simulink model "C28069_LLC_ePWM_V8_230307_PhaeShiftWorking"  (R2022b)
settings: Solver=FixedStepAuto  StartTime=0.0  StopTime=10  RelTol=1e-3  EnableMultiTasking=on
model workspace (MAT data in the model file):
  Comp_DAC = 512
undefined symbols (not defined in the file or in its folder): Down, GPTRIP1SEL, GPTRIP2SEL, PWM_Control, PWM_Gen, PWM_Gen1, SCI_A_Transmit, SCI_A_Transmit_Current_Suffix, SCI_A_Transmit_Duty_Suffix, SCI_A_Transmit_Freq_Suffix, SCI_A_Transmit_OVPFlag_Suffix, SCI_A_Transmit_PFC_Suffix, SCI_A_Transmit_SS_Suffix, SCI_A_Transmit_TBPHS_Suffix, SCI_A_Transmit_VADC_Suffix, SCI_A_Transmit_VAvg_Suffix, SCI_A_Transmit_VBAT_Suffix, SCI_A_Transmit_VBATRef_Suffix, SCI_A_Transmit_Vo_Suffix, TZ1, TZ2, u1, Up
libraries: c2802xlib x92, c280xlib x39, simulink x36, c2000lib x1
(part 3 of 18)

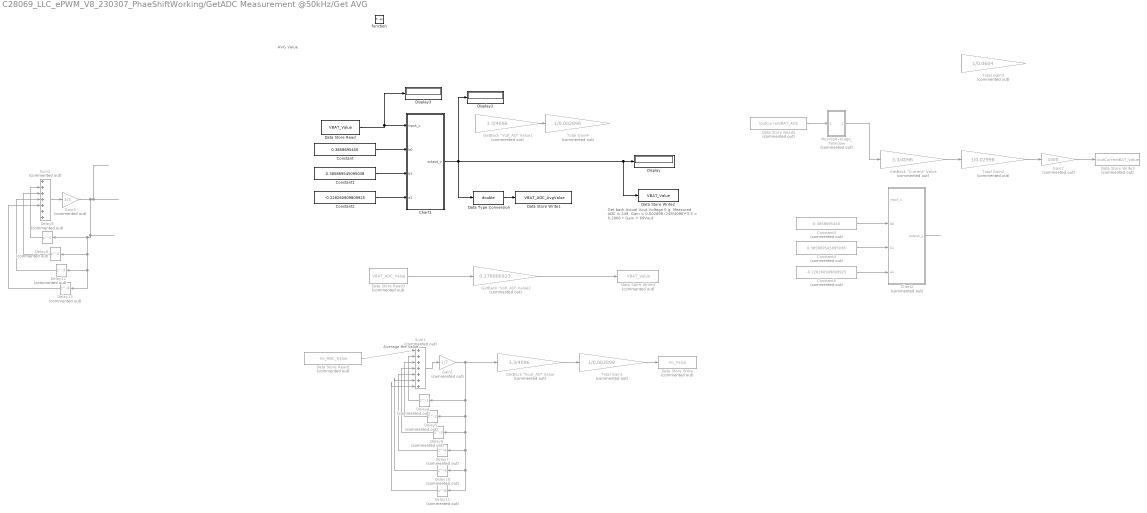
== system C28069_LLC_ePWM_V8_230307_PhaeShiftWorking/GetADC Measurement @50kHz/Get AVG ==
  note: AVG Value
  note: Average the value
  note: Get back Actual Vout Voltage
      | E.g.
      | Measured ADC is 249, Gain = 0.002898
      | (249/4096)*3.3 = 0.2006 * Gain
      | = 69Vout
  function : TriggerPort  TriggerType=function-call  VariantControl=(inherit)
  Chart1 : Stateflow chart  TreatAsAtomicUnit=on
  Chart2 : Stateflow chart  Commented=on  TreatAsAtomicUnit=on
  Constant : Constant  Value=0.3858695450
  Constant1 : Constant  Value=0.385869545095038
  Constant2 : Constant  Value=-0.228260909809925
  Constant3 : Constant  Commented=on  Value=0.3858695450
  Constant4 : Constant  Commented=on  Value=0.385869545095038
  Constant5 : Constant  Commented=on  Value=-0.228260909809925
  Data Store Read : DataStoreRead  DataStoreName=VBAT_Value  IndexOptions=Index vector (dialog)  Indices=1  OutputSizes=1
  Data Store Read1 : DataStoreRead  Commented=on  DataStoreName=Vo_ADC_Value  IndexOptions=Index vector (dialog)  Indices=1  OutputSizes=1
  Data Store Read2 : DataStoreRead  Commented=on  DataStoreName=IoutCurrentBAT_ADC  IndexOptions=Index vector (dialog)  Indices=1  OutputSizes=1
  Data Store Read3 : DataStoreRead  Commented=on  DataStoreName=VBAT_ADC_Value  IndexOptions=Index vector (dialog)  Indices=1  OutputSizes=1
  Data Store Write : DataStoreWrite  Commented=on  DataStoreName=Vo_Value  IndexOptions=Index vector (dialog)  Indices=1  OutputSizes=1
  Data Store Write1 : DataStoreWrite  DataStoreName=VBAT_ADC_AvgValue  IndexOptions=Index vector (dialog)  Indices=1  OutputSizes=1
  Data Store Write2 : DataStoreWrite  DataStoreName=VBAT_Value  IndexOptions=Index vector (dialog)  Indices=1  OutputSizes=1
  Data Store Write3 : DataStoreWrite  Commented=on  DataStoreName=IoutCurrentBAT_Value  IndexOptions=Index vector (dialog)  Indices=1  OutputSizes=1
  Data Store Write4 : DataStoreWrite  Commented=on  DataStoreName=VBAT_Value  IndexOptions=Index vector (dialog)  Indices=1  OutputSizes=1
  Data Type Conversion : DataTypeConversion  OutDataTypeStr=double  SaturateOnIntegerOverflow=off  RndMeth=Floor
  Delay10 : Delay  Commented=on  DelayLength=5
  Delay11 : Delay  Commented=on  DelayLength=6
  Delay12 : Delay  Commented=on  DelayLength=3
  Delay13 : Delay  Commented=on  DelayLength=4
  Delay4 : Delay  Commented=on  DelayLength=1
  Delay5 : Delay  Commented=on
  Delay6 : Delay  Commented=on  DelayLength=3
  Delay7 : Delay  Commented=on  DelayLength=4
  Delay8 : Delay  Commented=on  DelayLength=1
  Delay9 : Delay  Commented=on
  Display : Display
      settings: Decimation=2
  Display2 : Display
  Display3 : Display
  Gain1 : Gain  Commented=on  Gain=1/7  OutDataTypeStr=uint16
  Gain2 : Gain  Commented=on  Gain=1000
  Gain3 : Gain  Commented=on  Gain=1/5  OutDataTypeStr=uint16
  "GetBack \"Current\" Value" : Gain  Commented=on  Gain=3.3/4096  OutDataTypeStr=double
  "GetBack \"Volt_AD\" Value1" : Gain  Commented=on  Gain=3.3/4096  OutDataTypeStr=double
  "GetBack \"Volt_AD\" Value2" : Gain  Commented=on  Gain=0.278006923  OutDataTypeStr=double
  "GetBack \"Vout_AD\" Value" : Gain  Commented=on  Gain=3.3/4096  OutDataTypeStr=double
  MovingAverage_7Window : Subsystem  Commented=on
  Sum1 : Sum  Commented=on  Inputs=|+++++++
  Sum2 : Sum  Commented=on  Inputs=|+++++++
  Total Gain1 : Gain  Commented=on  Gain=1/0.002898  OutDataTypeStr=double
  Total Gain2 : Gain  Commented=on  Gain=1/0.02998  OutDataTypeStr=double
  Total Gain3 : Gain  Commented=on  Gain=1/0.0604  OutDataTypeStr=double
  Total Gain4 : Gain  Commented=on  Gain=1/0.002898  OutDataTypeStr=double
  wires:
  Delay4/1 -> Sum1/2
  Total Gain1/1 -> Data Store Write/1
  "GetBack \"Current\" Value"/1 -> Total Gain2/1
  Delay7/1 -> Sum1/5
  Gain1/1 -> Delay4/1, Delay5/1, Delay6/1, Delay7/1, Delay10/1, Delay11/1, "GetBack \"Vout_AD\" Value"/1
  Data Type Conversion/1 -> Data Store Write1/1
  Delay6/1 -> Sum1/4
  Delay11/1 -> Sum1/7
  Delay10/1 -> Sum1/6
  "GetBack \"Vout_AD\" Value"/1 -> Total Gain1/1
  Data Store Read1/1 -> Sum1/1
  Chart1/1(output_y) -> Display2/1, Display/1, Data Store Write2/1, Data Type Conversion/1
  Sum1/1 -> Gain1/1
  Delay5/1 -> Sum1/3
  Total Gain2/1 -> Gain2/1
  Gain2/1 -> Data Store Write3/1
  Gain3/1 -> Delay9/1, Delay12/1, Delay13/1, Delay8/1
  Delay9/1 -> Sum2/3
  Sum2/1 -> Gain3/1
  Delay13/1 -> Sum2/5
  Delay12/1 -> Sum2/4
  Delay8/1 -> Sum2/2
  Data Store Read/1 -> Display3/1, Chart1/1(input_u)
  Constant2/1 -> Chart1/4(a1)
  Constant1/1 -> Chart1/3(b1)
  Constant/1 -> Chart1/2(b0)
  Data Store Read2/1 -> MovingAverage_7Window/1(In1)
  Chart2/1(output_y) -> ?
  Constant5/1 -> Chart2/4(a1)
  Constant4/1 -> Chart2/3(b1)
  Constant3/1 -> Chart2/2(b0)
  MovingAverage_7Window/1(Out1) -> "GetBack \"Current\" Value"/1
  "GetBack \"Volt_AD\" Value1"/1 -> Total Gain4/1
  Data Store Read3/1 -> "GetBack \"Volt_AD\" Value2"/1
  "GetBack \"Volt_AD\" Value2"/1 -> Data Store Write4/1

== system C28069_LLC_ePWM_V8_230307_PhaeShiftWorking/GetADC Measurement @50kHz/MovingAverage_7Window ==
  note: Average the value
  In1 : Inport
  Delay12 : Delay  DelayLength=5
  Delay13 : Delay  DelayLength=6
  Delay14 : Delay  DelayLength=1
  Delay15 : Delay
  Delay16 : Delay  DelayLength=3
  Delay17 : Delay  DelayLength=4
  Gain2 : Gain  Gain=1/7  OutDataTypeStr=uint16
  Sum2 : Sum  Inputs=|+++++++
  Out1 : Outport
  wires:
  Delay17/1 -> Sum2/5
  Gain2/1 -> Out1/1, Delay13/1, Delay12/1, Delay17/1, Delay16/1, Delay15/1, Delay14/1
  In1/1 -> Sum2/1
  Delay12/1 -> Sum2/6
  Delay13/1 -> Sum2/7
  Delay16/1 -> Sum2/4
  Delay15/1 -> Sum2/3
  Delay14/1 -> Sum2/2
  Sum2/1 -> Gain2/1

== system C28069_LLC_ePWM_V8_230307_PhaeShiftWorking/GetADC, FaultProtection, SoftStart  @5KHz/Close Loop Regulation ==
  function : TriggerPort  TriggerType=function-call  VariantControl=(inherit)
  Constant : Constant
  Data Store Read1 : DataStoreRead  DataStoreName=SoftStart_OK_Signal  IndexOptions=Index vector (dialog)  Indices=1  OutputSizes=1
  Data Store Read4 : DataStoreRead  DataStoreName=PFC_OK  IndexOptions=Index vector (dialog)  Indices=1  OutputSizes=1
  If : If  NumInputs=2  IfExpression=(u1 == 1) & (u2 == 1)  ShowElse=off
  If Action Subsystem : Subsystem  TreatAsAtomicUnit=on
  wires:
  Constant/1 -> If/2
  If/1 -> If Action Subsystem/Action
  Data Store Read4/1 -> If/1

== system C28069_LLC_ePWM_V8_230307_PhaeShiftWorking/GetADC, FaultProtection, SoftStart  @5KHz/Fault Protection @ 5KHz ==
  function : TriggerPort  TriggerType=function-call  VariantControl=(inherit)
  Data Store Read4 : DataStoreRead  DataStoreName=PFC_OK  IndexOptions=Index vector (dialog)  Indices=1  OutputSizes=1
  If : If  IfExpression=u1 == 1  ShowElse=off
  If Action Subsystem : Subsystem  Commented=on  TreatAsAtomicUnit=on
  wires:
  If/1 -> If Action Subsystem/Action
  Data Store Read4/1 -> If/1

== system C28069_LLC_ePWM_V8_230307_PhaeShiftWorking/GetADC, FaultProtection, SoftStart  @5KHz/Fault Protection @ 5KHz1 ==
  function : TriggerPort  TriggerType=function-call  VariantControl=(inherit)
  Data Store Read4 : DataStoreRead  DataStoreName=PFC_OK  IndexOptions=Index vector (dialog)  Indices=1  OutputSizes=1
  If : If  IfExpression=u1 == 1  ShowElse=off
  If Action Subsystem : Subsystem  Commented=on  TreatAsAtomicUnit=on
  wires:
  If/1 -> If Action Subsystem/Action
  Data Store Read4/1 -> If/1

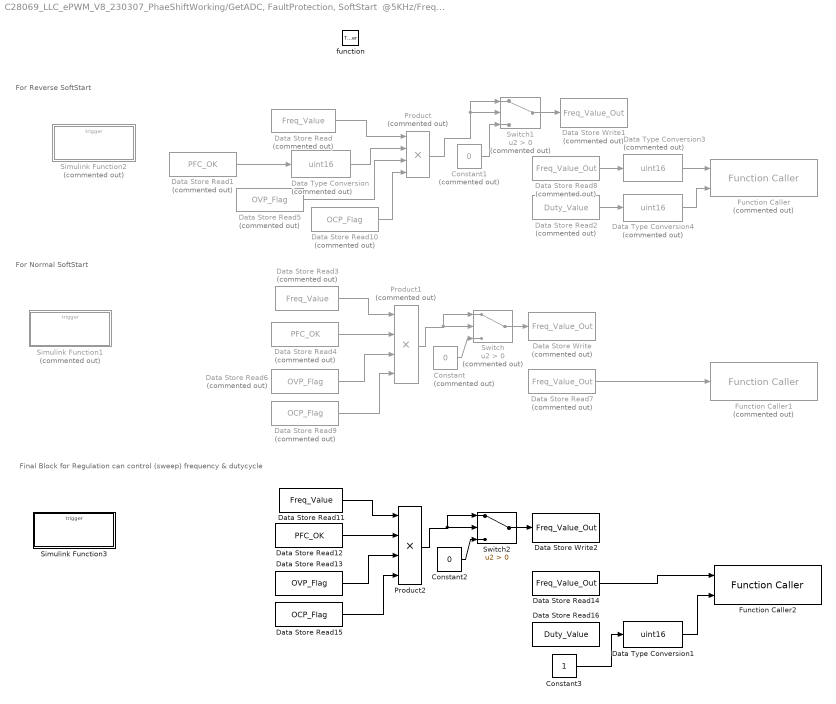
== system C28069_LLC_ePWM_V8_230307_PhaeShiftWorking/GetADC, FaultProtection, SoftStart  @5KHz/Frequency Update ==
  note: For Reverse SoftStart
  note: For Normal SoftStart
  note: Final Block for Regulation can control (sweep) frequency & dutycycle
  function : TriggerPort  TriggerType=function-call  VariantControl=(inherit)
  Constant : Constant  Commented=on  Value=0  OutDataTypeStr=double
  Constant1 : Constant  Commented=on  Value=0
  Constant2 : Constant  Value=0  OutDataTypeStr=double
  Constant3 : Constant  OutDataTypeStr=double
  Data Store Read : DataStoreRead  Commented=on  DataStoreName=Freq_Value  IndexOptions=Index vector (dialog)  Indices=1  OutputSizes=1
  Data Store Read1 : DataStoreRead  Commented=on  DataStoreName=PFC_OK  IndexOptions=Index vector (dialog)  Indices=1  OutputSizes=1
  Data Store Read10 : DataStoreRead  Commented=on  DataStoreName=OCP_Flag  IndexOptions=Index vector (dialog)  Indices=1  OutputSizes=1
  Data Store Read11 : DataStoreRead  DataStoreName=Freq_Value  IndexOptions=Index vector (dialog)  Indices=1  OutputSizes=1
  Data Store Read12 : DataStoreRead  DataStoreName=PFC_OK  IndexOptions=Index vector (dialog)  Indices=1  OutputSizes=1
  Data Store Read13 : DataStoreRead  DataStoreName=OVP_Flag  IndexOptions=Index vector (dialog)  Indices=1  OutputSizes=1
  Data Store Read14 : DataStoreRead  DataStoreName=Freq_Value_Out  IndexOptions=Index vector (dialog)  Indices=1  OutputSizes=1
  Data Store Read15 : DataStoreRead  DataStoreName=OCP_Flag  IndexOptions=Index vector (dialog)  Indices=1  OutputSizes=1
  Data Store Read16 : DataStoreRead  DataStoreName=Duty_Value  IndexOptions=Index vector (dialog)  Indices=1  OutputSizes=1
  Data Store Read2 : DataStoreRead  Commented=on  DataStoreName=Duty_Value  IndexOptions=Index vector (dialog)  Indices=1  OutputSizes=1
  Data Store Read3 : DataStoreRead  Commented=on  DataStoreName=Freq_Value  IndexOptions=Index vector (dialog)  Indices=1  OutputSizes=1
  Data Store Read4 : DataStoreRead  Commented=on  DataStoreName=PFC_OK  IndexOptions=Index vector (dialog)  Indices=1  OutputSizes=1
  Data Store Read5 : DataStoreRead  Commented=on  DataStoreName=OVP_Flag  IndexOptions=Index vector (dialog)  Indices=1  OutputSizes=1
  Data Store Read6 : DataStoreRead  Commented=on  DataStoreName=OVP_Flag  IndexOptions=Index vector (dialog)  Indices=1  OutputSizes=1
  Data Store Read7 : DataStoreRead  Commented=on  DataStoreName=Freq_Value_Out  IndexOptions=Index vector (dialog)  Indices=1  OutputSizes=1
  Data Store Read8 : DataStoreRead  Commented=on  DataStoreName=Freq_Value_Out  IndexOptions=Index vector (dialog)  Indices=1  OutputSizes=1
  Data Store Read9 : DataStoreRead  Commented=on  DataStoreName=OCP_Flag  IndexOptions=Index vector (dialog)  Indices=1  OutputSizes=1
  Data Store Write : DataStoreWrite  Commented=on  DataStoreName=Freq_Value_Out  IndexOptions=Index vector (dialog)  Indices=1  OutputSizes=1
  Data Store Write1 : DataStoreWrite  Commented=on  DataStoreName=Freq_Value_Out  IndexOptions=Index vector (dialog)  Indices=1  OutputSizes=1
  Data Store Write2 : DataStoreWrite  DataStoreName=Freq_Value_Out  IndexOptions=Index vector (dialog)  Indices=1  OutputSizes=1
  Data Type Conversion : DataTypeConversion  Commented=on  OutDataTypeStr=uint16  SaturateOnIntegerOverflow=off  RndMeth=Floor
  Data Type Conversion1 : DataTypeConversion  OutDataTypeStr=uint16  SaturateOnIntegerOverflow=off  RndMeth=Floor
  Data Type Conversion3 : DataTypeConversion  Commented=on  OutDataTypeStr=uint16  SaturateOnIntegerOverflow=off  RndMeth=Floor
  Data Type Conversion4 : DataTypeConversion  Commented=on  OutDataTypeStr=uint16  SaturateOnIntegerOverflow=off  RndMeth=Floor
  Function Caller : FunctionCaller  Commented=on  FunctionPrototype=PWM_Gen1(u,u1)  InputArgumentSpecifications=<Enter example>  OutputArgumentSpecifications=<Enter example>
  Function Caller1 : FunctionCaller  Commented=on  FunctionPrototype=PWM_Gen(u)  InputArgumentSpecifications=<Enter example>  OutputArgumentSpecifications=<Enter example>
  Function Caller2 : FunctionCaller  FunctionPrototype=PWM_Control(u,u1)  InputArgumentSpecifications=<Enter example>  OutputArgumentSpecifications=<Enter example>
  Product : Product  Commented=on  Inputs=4  OutDataTypeStr=uint16
  Product1 : Product  Commented=on  Inputs=4  OutDataTypeStr=double
  Product2 : Product  Inputs=4  OutDataTypeStr=double
  Simulink Function1 : Subsystem  Commented=on  TreatAsAtomicUnit=on
  Simulink Function2 : Subsystem  Commented=on  TreatAsAtomicUnit=on
  Simulink Function3 : Subsystem  TreatAsAtomicUnit=on
  Switch : Switch  Commented=on  Criteria=u2 > Threshold  OutDataTypeStr=double  SaturateOnIntegerOverflow=off  InputSameDT=off
  Switch1 : Switch  Commented=on  Criteria=u2 > Threshold  SaturateOnIntegerOverflow=off  InputSameDT=off
  Switch2 : Switch  Criteria=u2 > Threshold  OutDataTypeStr=double  SaturateOnIntegerOverflow=off  InputSameDT=off
  wires:
  Data Store Read1/1 -> Data Type Conversion/1
  Data Type Conversion/1 -> Product/2
  Data Store Read7/1 -> Function Caller1/1
  Product1/1 -> Switch/2, Switch/1
  Data Store Read2/1 -> Data Type Conversion4/1
  Data Store Read10/1 -> Product/4
  Data Store Read5/1 -> Product/3
  Constant1/1 -> Switch1/3
  Data Store Read4/1 -> Product1/2
  Data Store Read/1 -> Product/1
  Product/1 -> Switch1/2, Switch1/1
  Data Store Read9/1 -> Product1/4
  Constant/1 -> Switch/3
  Data Type Conversion3/1 -> Function Caller/1
  Data Store Read6/1 -> Product1/3
  Switch1/1 -> Data Store Write1/1
  Switch/1 -> Data Store Write/1
  Data Type Conversion4/1 -> Function Caller/2
  Data Store Read3/1 -> Product1/1
  Data Store Read8/1 -> Data Type Conversion3/1
  Constant2/1 -> Switch2/3
  Data Store Read11/1 -> Product2/1
  Switch2/1 -> Data Store Write2/1
  Data Store Read15/1 -> Product2/4
  Data Store Read13/1 -> Product2/3
  Product2/1 -> Switch2/2, Switch2/1
  Data Store Read12/1 -> Product2/2
  Data Store Read14/1 -> Function Caller2/1
  Data Type Conversion1/1 -> Function Caller2/2
  Constant3/1 -> Data Type Conversion1/1

== system C28069_LLC_ePWM_V8_230307_PhaeShiftWorking/GetADC, FaultProtection, SoftStart  @5KHz/Get AVG ==
  note: Get back Actual Vout Voltage
      | E.g.
      | Measured ADC is 249, Gain = 0.002898
      | (249/4096)*3.3 = 0.2006 * Gain
      | = 69Vout
  note: AVG Value
  note: Average the value
  function : TriggerPort  TriggerType=function-call  VariantControl=(inherit)
  Constant : Constant  Value=249
  Data Store Read : DataStoreRead  DataStoreName=VBAT_ADC_Value  IndexOptions=Index vector (dialog)  Indices=1  OutputSizes=1
  Data Store Read1 : DataStoreRead  DataStoreName=Vo_ADC_Value  IndexOptions=Index vector (dialog)  Indices=1  OutputSizes=1
  Data Store Read2 : DataStoreRead  DataStoreName=IoutCurrentBAT_ADC  IndexOptions=Index vector (dialog)  Indices=1  OutputSizes=1
  Data Store Write : DataStoreWrite  DataStoreName=Vo_Value  IndexOptions=Index vector (dialog)  Indices=1  OutputSizes=1
  Data Store Write1 : DataStoreWrite  DataStoreName=VBAT_ADC_AvgValue  IndexOptions=Index vector (dialog)  Indices=1  OutputSizes=1
  Data Store Write2 : DataStoreWrite  DataStoreName=VBAT_Value  IndexOptions=Index vector (dialog)  Indices=1  OutputSizes=1
  Data Store Write3 : DataStoreWrite  DataStoreName=IoutCurrentBAT_Value  IndexOptions=Index vector (dialog)  Indices=1  OutputSizes=1
  Data Type Conversion : DataTypeConversion  OutDataTypeStr=double  SaturateOnIntegerOverflow=off  RndMeth=Floor
  Delay : Delay  DelayLength=1
  Delay1 : Delay
  Delay10 : Delay  DelayLength=5
  Delay11 : Delay  DelayLength=6
  Delay2 : Delay  DelayLength=3
  Delay3 : Delay  DelayLength=4
  Delay4 : Delay  DelayLength=1
  Delay5 : Delay
  Delay6 : Delay  DelayLength=3
  Delay7 : Delay  DelayLength=4
  Display : Display
      settings: Decimation=2
  Display2 : Display
  Display3 : Display
  Gain : Gain  Gain=1/5  OutDataTypeStr=uint16
  Gain1 : Gain  Gain=1/7  OutDataTypeStr=uint16
  Gain2 : Gain  Gain=1000
  "GetBack \"Current\" Value" : Gain  Gain=3.3/4096  OutDataTypeStr=double
  "GetBack \"Volt_AD\" Value" : Gain  Gain=3.3/4096  OutDataTypeStr=double
  "GetBack \"Vout_AD\" Value" : Gain  Gain=3.3/4096  OutDataTypeStr=double
  MovingAverage_7Window : Subsystem
  Sum : Sum  Inputs=|+++++++
  Sum1 : Sum  Inputs=|+++++++
  Total Gain : Gain  Gain=1/0.002898  OutDataTypeStr=double
  Total Gain1 : Gain  Gain=1/0.002898  OutDataTypeStr=double
  Total Gain2 : Gain  Gain=1/0.02998  OutDataTypeStr=double
  Total Gain3 : Gain  Commented=on  Gain=1/0.0604  OutDataTypeStr=double
  wires:
  Delay1/1 -> Sum/3
  Data Store Read/1 -> Sum/1, Display3/1
  Total Gain/1 -> Data Store Write2/1, Display/1
  Delay/1 -> Sum/2
  Delay2/1 -> Sum/4
  "GetBack \"Volt_AD\" Value"/1 -> Total Gain/1
  Delay3/1 -> Sum/5
  Data Type Conversion/1 -> Data Store Write1/1
  "GetBack \"Vout_AD\" Value"/1 -> Total Gain1/1
  Total Gain1/1 -> Data Store Write/1
  Delay11/1 -> Sum1/7
  Delay10/1 -> Sum1/6
  Gain1/1 -> "GetBack \"Vout_AD\" Value"/1, Delay11/1, Delay10/1, Delay7/1, Delay6/1, Delay5/1, Delay4/1
  Sum1/1 -> Gain1/1
  Delay7/1 -> Sum1/5
  Delay6/1 -> Sum1/4
  Delay5/1 -> Sum1/3
  Delay4/1 -> Sum1/2
  Data Store Read1/1 -> Sum1/1
  Data Store Read2/1 -> MovingAverage_7Window/1(In1)
  MovingAverage_7Window/1(Out1) -> "GetBack \"Current\" Value"/1
  "GetBack \"Current\" Value"/1 -> Total Gain2/1
  Total Gain2/1 -> Gain2/1
  Gain2/1 -> Data Store Write3/1
  Sum/1 -> Gain/1
  Gain/1 -> Data Type Conversion/1, "GetBack \"Volt_AD\" Value"/1, Display2/1, Delay/1, Delay3/1, Delay2/1, Delay1/1

== system C28069_LLC_ePWM_V8_230307_PhaeShiftWorking/GetADC, FaultProtection, SoftStart  @5KHz/Get AVG1 ==
  note: AVG Value
  note: Get back Actual Vout Voltage
      | E.g.
      | Measured ADC is 249, Gain = 0.002898
      | (249/4096)*3.3 = 0.2006 * Gain
      | = 69Vout
  note: Average the value
  Action Port : ActionPort  ActionPortLabel=case [ 1 ]:
  Constant : Constant  Value=249
  Data Store Read : DataStoreRead  DataStoreName=VBAT_ADC_Value  IndexOptions=Index vector (dialog)  Indices=1  OutputSizes=1
  Data Store Read1 : DataStoreRead  DataStoreName=Vo_ADC_Value  IndexOptions=Index vector (dialog)  Indices=1  OutputSizes=1
  Data Store Read2 : DataStoreRead  DataStoreName=IoutCurrentBAT_ADC  IndexOptions=Index vector (dialog)  Indices=1  OutputSizes=1
  Data Store Write : DataStoreWrite  DataStoreName=Vo_Value  IndexOptions=Index vector (dialog)  Indices=1  OutputSizes=1
  Data Store Write1 : DataStoreWrite  DataStoreName=VBAT_ADC_AvgValue  IndexOptions=Index vector (dialog)  Indices=1  OutputSizes=1
  Data Store Write2 : DataStoreWrite  DataStoreName=VBAT_Value  IndexOptions=Index vector (dialog)  Indices=1  OutputSizes=1
  Data Store Write3 : DataStoreWrite  DataStoreName=IoutCurrentBAT_Value  IndexOptions=Index vector (dialog)  Indices=1  OutputSizes=1
  Data Type Conversion : DataTypeConversion  OutDataTypeStr=double  SaturateOnIntegerOverflow=off  RndMeth=Floor
  Delay : Delay  DelayLength=1
  Delay1 : Delay
  Delay10 : Delay  DelayLength=5
  Delay11 : Delay  DelayLength=6
  Delay2 : Delay  DelayLength=3
  Delay3 : Delay  DelayLength=4
  Delay4 : Delay  DelayLength=1
  Delay5 : Delay
  Delay6 : Delay  DelayLength=3
  Delay7 : Delay  DelayLength=4
  Display : Display
      settings: Decimation=2
  Display2 : Display
  Display3 : Display
  Gain : Gain  Gain=1/5  OutDataTypeStr=uint16
  Gain1 : Gain  Gain=1/7  OutDataTypeStr=uint16
  Gain2 : Gain  Gain=1000
  "GetBack \"Current\" Value" : Gain  Gain=3.3/4096  OutDataTypeStr=double
  "GetBack \"Volt_AD\" Value" : Gain  Gain=3.3/4096  OutDataTypeStr=double
  "GetBack \"Vout_AD\" Value" : Gain  Gain=3.3/4096  OutDataTypeStr=double
  MovingAverage_7Window : Subsystem
  Sum : Sum  Inputs=|+++++++
  Sum1 : Sum  Inputs=|+++++++
  Total Gain : Gain  Gain=1/0.002898  OutDataTypeStr=double
  Total Gain1 : Gain  Gain=1/0.002898  OutDataTypeStr=double
  Total Gain2 : Gain  Gain=1/0.02998  OutDataTypeStr=double
  Total Gain3 : Gain  Commented=on  Gain=1/0.0604  OutDataTypeStr=double
  wires:
  Data Store Read/1 -> Display3/1, Sum/1
  Delay7/1 -> Sum1/5
  Gain1/1 -> Delay4/1, Delay5/1, Delay6/1, Delay7/1, Delay10/1, Delay11/1, "GetBack \"Vout_AD\" Value"/1
  Total Gain1/1 -> Data Store Write/1
  Sum1/1 -> Gain1/1
  Delay5/1 -> Sum1/3
  Delay4/1 -> Sum1/2
  Delay1/1 -> Sum/3
  "GetBack \"Current\" Value"/1 -> Total Gain2/1
  Data Type Conversion/1 -> Data Store Write1/1
  Total Gain/1 -> Display/1, Data Store Write2/1
  Delay2/1 -> Sum/4
  "GetBack \"Volt_AD\" Value"/1 -> Total Gain/1
  Delay/1 -> Sum/2
  Delay3/1 -> Sum/5
  Data Store Read1/1 -> Sum1/1
  Delay6/1 -> Sum1/4
  Delay10/1 -> Sum1/6
  MovingAverage_7Window/1(Out1) -> "GetBack \"Current\" Value"/1
  Data Store Read2/1 -> MovingAverage_7Window/1(In1)
  Gain/1 -> Delay1/1, Delay2/1, Delay3/1, Delay/1, Display2/1, "GetBack \"Volt_AD\" Value"/1, Data Type Conversion/1
  Delay11/1 -> Sum1/7
  Sum/1 -> Gain/1
  Total Gain2/1 -> Gain2/1
  "GetBack \"Vout_AD\" Value"/1 -> Total Gain1/1
  Gain2/1 -> Data Store Write3/1

== system C28069_LLC_ePWM_V8_230307_PhaeShiftWorking/GetADC, FaultProtection, SoftStart  @5KHz/Get AVG2 ==
  note: AVG Value
  note: Average the value
  note: Get back Actual Vout Voltage
      | E.g.
      | Measured ADC is 249, Gain = 0.002898
      | (249/4096)*3.3 = 0.2006 * Gain
      | = 69Vout
  function : TriggerPort  TriggerType=function-call  VariantControl=(inherit)
  Constant : Constant  Value=249
  Data Store Read : DataStoreRead  DataStoreName=VBAT_ADC_Value  IndexOptions=Index vector (dialog)  Indices=1  OutputSizes=1
  Data Store Read1 : DataStoreRead  DataStoreName=Vo_ADC_Value  IndexOptions=Index vector (dialog)  Indices=1  OutputSizes=1
  Data Store Read2 : DataStoreRead  DataStoreName=IoutCurrentBAT_ADC  IndexOptions=Index vector (dialog)  Indices=1  OutputSizes=1
  Data Store Write : DataStoreWrite  DataStoreName=Vo_Value  IndexOptions=Index vector (dialog)  Indices=1  OutputSizes=1
  Data Store Write1 : DataStoreWrite  DataStoreName=VBAT_ADC_AvgValue  IndexOptions=Index vector (dialog)  Indices=1  OutputSizes=1
  Data Store Write2 : DataStoreWrite  DataStoreName=VBAT_Value  IndexOptions=Index vector (dialog)  Indices=1  OutputSizes=1
  Data Store Write3 : DataStoreWrite  DataStoreName=IoutCurrentBAT_Value  IndexOptions=Index vector (dialog)  Indices=1  OutputSizes=1
  Data Type Conversion : DataTypeConversion  OutDataTypeStr=double  SaturateOnIntegerOverflow=off  RndMeth=Floor
  Delay : Delay  DelayLength=1
  Delay1 : Delay
  Delay10 : Delay  DelayLength=5
  Delay11 : Delay  DelayLength=6
  Delay2 : Delay  DelayLength=3
  Delay3 : Delay  DelayLength=4
  Delay4 : Delay  DelayLength=1
  Delay5 : Delay
  Delay6 : Delay  DelayLength=3
  Delay7 : Delay  DelayLength=4
  Display : Display
      settings: Decimation=2
  Display2 : Display
  Display3 : Display
  Gain : Gain  Gain=1/5  OutDataTypeStr=uint16
  Gain1 : Gain  Gain=1/7  OutDataTypeStr=uint16
  Gain2 : Gain  Gain=1000
  "GetBack \"Current\" Value" : Gain  Gain=3.3/4096  OutDataTypeStr=double
  "GetBack \"Volt_AD\" Value" : Gain  Gain=3.3/4096  OutDataTypeStr=double
  "GetBack \"Vout_AD\" Value" : Gain  Gain=3.3/4096  OutDataTypeStr=double
  MovingAverage_7Window : Subsystem
  Sum : Sum  Inputs=|+++++++
  Sum1 : Sum  Inputs=|+++++++
  Total Gain : Gain  Gain=1/0.002898  OutDataTypeStr=double
  Total Gain1 : Gain  Gain=1/0.002898  OutDataTypeStr=double
  Total Gain2 : Gain  Gain=1/0.02998  OutDataTypeStr=double
  Total Gain3 : Gain  Commented=on  Gain=1/0.0604  OutDataTypeStr=double
  wires:
  Delay4/1 -> Sum1/2
  Delay1/1 -> Sum/3
  Total Gain1/1 -> Data Store Write/1
  "GetBack \"Current\" Value"/1 -> Total Gain2/1
  Delay7/1 -> Sum1/5
  Gain1/1 -> Delay4/1, Delay5/1, Delay6/1, Delay7/1, Delay10/1, Delay11/1, "GetBack \"Vout_AD\" Value"/1
  Data Type Conversion/1 -> Data Store Write1/1
  Delay6/1 -> Sum1/4
  Gain/1 -> Delay1/1, Delay2/1, Delay3/1, Delay/1, Display2/1, "GetBack \"Volt_AD\" Value"/1, Data Type Conversion/1
  Data Store Read2/1 -> MovingAverage_7Window/1(In1)
  Delay3/1 -> Sum/5
  Delay11/1 -> Sum1/7
  Delay10/1 -> Sum1/6
  Data Store Read/1 -> Display3/1, Sum/1
  "GetBack \"Vout_AD\" Value"/1 -> Total Gain1/1
  "GetBack \"Volt_AD\" Value"/1 -> Total Gain/1
  Data Store Read1/1 -> Sum1/1
  Total Gain/1 -> Display/1, Data Store Write2/1
  Delay/1 -> Sum/2
  Sum/1 -> Gain/1
  Sum1/1 -> Gain1/1
  Delay5/1 -> Sum1/3
  MovingAverage_7Window/1(Out1) -> "GetBack \"Current\" Value"/1
  Total Gain2/1 -> Gain2/1
  Gain2/1 -> Data Store Write3/1
  Delay2/1 -> Sum/4

== system C28069_LLC_ePWM_V8_230307_PhaeShiftWorking/GetADC, FaultProtection, SoftStart  @5KHz/SoftStart ==
  function : TriggerPort  TriggerType=function-call  VariantControl=(inherit)
  Data Store Read1 : DataStoreRead  DataStoreName=SoftStart_OK_Signal  IndexOptions=Index vector (dialog)  Indices=1  OutputSizes=1
  If : If  IfExpression=u1 == 0  ShowElse=off
  If Action Subsystem : Subsystem  TreatAsAtomicUnit=on
  wires:
  Data Store Read1/1 -> If/1
  If/1 -> If Action Subsystem/Action

== system C28069_LLC_ePWM_V8_230307_PhaeShiftWorking/GetADC, FaultProtection, SoftStart  @5KHz/SoftStart1 ==
  function : TriggerPort  TriggerType=function-call  VariantControl=(inherit)
  Data Store Read1 : DataStoreRead  DataStoreName=SoftStart_OK_Signal  IndexOptions=Index vector (dialog)  Indices=1  OutputSizes=1
  Function-Call Generator : simulink/Ports & Subsystems/Function-Call Generator  Commented=on  sample_time=-1  numberOfIterations=1  DisallowWideOutput=off
  Function-Call Split : FunctionCallSplit  Commented=on  IconShape=distinctive  NumOutputPorts=2  OutputPortLayout=default
  If : If  IfExpression=u1 == 0  ShowElse=off
  If Action Subsystem : Subsystem  TreatAsAtomicUnit=on
  ReservseSoftStart : Subsystem  Commented=on  TreatAsAtomicUnit=on
  SoftStart : Subsystem  Commented=on  TreatAsAtomicUnit=on
  wires:
  If/1 -> If Action Subsystem/Action
  Data Store Read1/1 -> If/1
  Function-Call Split/1 -> SoftStart/Trigger
  Function-Call Split/2 -> ReservseSoftStart/Trigger
  Function-Call Generator/1 -> Function-Call Split/1

== system C28069_LLC_ePWM_V8_230307_PhaeShiftWorking/GetADC, FaultProtection, SoftStart  @5KHz/UpdatePWM ==
  function : TriggerPort  TriggerType=function-call  VariantControl=(inherit)
  Close Loop Regulation : Subsystem  TreatAsAtomicUnit=on
  Frequency Update : Subsystem  TreatAsAtomicUnit=on
  Function-Call Generator : simulink/Ports & Subsystems/Function-Call Generator  sample_time=-1  numberOfIterations=1  DisallowWideOutput=off
  Function-Call Split : FunctionCallSplit  IconShape=distinctive  NumOutputPorts=3  OutputPortLayout=default
  wires:
  Function-Call Generator/1 -> Function-Call Split/1
  Function-Call Split/2 -> Frequency Update/Trigger
  Function-Call Split/1 -> Close Loop Regulation/Trigger

== system C28069_LLC_ePWM_V8_230307_PhaeShiftWorking/GetADC, FaultProtection, SoftStart  @5KHz/UpdatePWM1 ==
  Action Port : ActionPort  ActionPortLabel=case [ 2 ]:
  Close Loop Regulation : Subsystem  TreatAsAtomicUnit=on
  Frequency Update : Subsystem  TreatAsAtomicUnit=on
  Function-Call Generator : simulink/Ports & Subsystems/Function-Call Generator  sample_time=-1  numberOfIterations=1  DisallowWideOutput=off
  Function-Call Split : FunctionCallSplit  IconShape=distinctive  NumOutputPorts=3  OutputPortLayout=default
  SoftStart : Subsystem  TreatAsAtomicUnit=on
  wires:
  Function-Call Generator/1 -> Function-Call Split/1
  Function-Call Split/3 -> Frequency Update/Trigger
  Function-Call Split/2 -> Close Loop Regulation/Trigger
  Function-Call Split/1 -> SoftStart/Trigger

== system C28069_LLC_ePWM_V8_230307_PhaeShiftWorking/Initialize Function1/Subsystem1 ==
  note: DutyCycle
  note: Frequency(kHz)
  freq : Inport
  duty : Inport  Port=2
  Constant2 : Constant  Value=90E6  OutDataTypeStr=uint32
  Constant3 : Constant  OutDataTypeStr=uint32
  Constant5 : Constant  Value=2  OutDataTypeStr=uint32
  Constant7 : Constant  Value=100
  Divide1 : Product  Inputs=*/  OutDataTypeStr=uint32
  Divide3 : Product  Inputs=*/
  Gain : Gain  Gain=1000
  Product1 : Product  OutDataTypeStr=uint32
  Product3 : Product  OutDataTypeStr=uint32
  Subtract1 : Sum  Inputs=+-
  Out1 : Outport
  Out2 : Outport  Port=2
  wires:
  Constant7/1 -> Divide3/2
  Constant5/1 -> Product3/2
  Constant3/1 -> Subtract1/1
  Divide3/1 -> Subtract1/2
  Subtract1/1 -> Product1/1
  Product3/1 -> Divide1/2
  Divide1/1 -> Out1/1, Product1/2
  Constant2/1 -> Divide1/1
  freq/1 -> Gain/1
  Product1/1 -> Out2/1
  duty/1 -> Divide3/1
  Gain/1 -> Product3/1

== system C28069_LLC_ePWM_V8_230307_PhaeShiftWorking/Initialize Function1/Subsystem2 ==
  note: DutyCycle
  note: Frequency(kHz)
  freq : Inport
  duty : Inport  Port=2
  Constant2 : Constant  Value=90E6  OutDataTypeStr=uint32
  Constant3 : Constant  OutDataTypeStr=uint32
  Constant5 : Constant  Value=2  OutDataTypeStr=uint32
  Constant7 : Constant  Value=100
  Divide1 : Product  Inputs=*/  OutDataTypeStr=uint32
  Divide3 : Product  Inputs=*/
  Gain : Gain  Gain=1000
  Product1 : Product  OutDataTypeStr=uint32
  Product3 : Product  OutDataTypeStr=uint32
  Subtract1 : Sum  Inputs=+-
  Out1 : Outport
  Out2 : Outport  Port=2
  wires:
  Constant7/1 -> Divide3/2
  Constant5/1 -> Product3/2
  Constant3/1 -> Subtract1/1
  Divide3/1 -> Subtract1/2
  Subtract1/1 -> Product1/1
  Product3/1 -> Divide1/2
  Divide1/1 -> Out1/1, Product1/2
  Constant2/1 -> Divide1/1
  freq/1 -> Gain/1
  Product1/1 -> Out2/1
  duty/1 -> Divide3/1
  Gain/1 -> Product3/1

== system C28069_LLC_ePWM_V8_230307_PhaeShiftWorking/Initialize Function1/Subsystem3 ==
  note: DutyCycle
  note: Frequency(kHz)
  freq : Inport
  duty : Inport  Port=2
  Constant2 : Constant  Value=90E6  OutDataTypeStr=uint32
  Constant3 : Constant  OutDataTypeStr=uint32
  Constant5 : Constant  Value=2  OutDataTypeStr=uint32
  Constant7 : Constant  Value=100
  Divide1 : Product  Inputs=*/  OutDataTypeStr=uint32
  Divide3 : Product  Inputs=*/
  Gain : Gain  Gain=1000
  Product1 : Product  OutDataTypeStr=uint32
  Product3 : Product  OutDataTypeStr=uint32
  Subtract1 : Sum  Inputs=+-
  Out1 : Outport
  Out2 : Outport  Port=2
  wires:
  Constant7/1 -> Divide3/2
  Constant5/1 -> Product3/2
  Constant3/1 -> Subtract1/1
  Divide3/1 -> Subtract1/2
  Subtract1/1 -> Product1/1
  Product3/1 -> Divide1/2
  Divide1/1 -> Out1/1, Product1/2
  Constant2/1 -> Divide1/1
  freq/1 -> Gain/1
  Product1/1 -> Out2/1
  duty/1 -> Divide3/1
  Gain/1 -> Product3/1

== system C28069_LLC_ePWM_V8_230307_PhaeShiftWorking/Initialize Function1/Subsystem4 ==
  Hz : Inport
  Duty : Inport  Port=2
  128*14 divider : Gain  Gain=1/(128*14)
  Constant1 : Constant  Value=90E6
  Constant2 : Constant
  Divide : Product  Inputs=*/  RndMeth=Zero  SaturateOnIntegerOverflow=on
  Floor : Rounding  Operator=round
  Floor1 : Rounding  Operator=round
  Gain1 : Gain  Gain=1/100
  Product1 : Product
  Subtract : Sum  Inputs=+-
  Out1 : Outport
  Out2 : Outport  Port=2
  wires:
  Duty/1 -> Gain1/1
  Divide/1 -> Floor/1, Product1/1
  Floor1/1 -> Out2/1
  Hz/1 -> 128*14 divider/1
  128*14 divider/1 -> Divide/2
  Constant2/1 -> Subtract/1
  Gain1/1 -> Subtract/2
  Constant1/1 -> Divide/1
  Subtract/1 -> Product1/2
  Product1/1 -> Floor1/1
  Floor/1 -> Out1/1

== system C28069_LLC_ePWM_V8_230307_PhaeShiftWorking/PFC_OK via UART1/Function-Call Subsystem ==
  function : TriggerPort  TriggerType=function-call  VariantControl=(inherit)
  Constant : Constant  Value=0
  Constant1 : Constant
  Data Store Write : DataStoreWrite  Commented=on  DataStoreName=PWM_Freq  IndexOptions=Index vector (dialog)  Indices=1  OutputSizes=1
  Data Store Write1 : DataStoreWrite  DataStoreName=PFC_OK  IndexOptions=Index vector (dialog)  Indices=1  OutputSizes=1
  Function Caller : FunctionCaller  Commented=on  FunctionPrototype=y = SCI_Receive()  InputArgumentSpecifications=<Enter example>  OutputArgumentSpecifications=<Enter example>
  Function Caller2 : FunctionCaller  FunctionPrototype=y = SCI_Receive()  InputArgumentSpecifications=<Enter example>  OutputArgumentSpecifications=<Enter example>
  Switch : Switch  Criteria=u2 > Threshold  SaturateOnIntegerOverflow=off  InputSameDT=off
  wires:
  Function Caller/1 -> Data Store Write/1
  Switch/1 -> Data Store Write1/1
  Function Caller2/1 -> Switch/2
  Constant/1 -> Switch/3
  Constant1/1 -> Switch/1

== system C28069_LLC_ePWM_V8_230307_PhaeShiftWorking/PFC_OK via UART1/Function-Call Subsystem1 ==
  note: PFC_OK = 1 = Enable PWM
  function : TriggerPort  TriggerType=function-call  VariantControl=(inherit)

== system C28069_LLC_ePWM_V8_230307_PhaeShiftWorking/PFC_OK via UART1/Simulink Function ==
  SCI_Receive : TriggerPort  TriggerType=function-call  IsSimulinkFunction=on  FunctionName=SCI_Receive  FunctionVisibility=scoped  VariantControl=(inherit)
  Constant2 : Constant  Value=48
  Constant3 : Constant  Value=48
  Constant4 : Constant  Value=48
  Demux : Demux  Outputs=3
  Gain2 : Gain  Gain=100
  Gain3 : Gain  Gain=10
  Gain4 : Gain
  SCI B Receive : c280xlib/SCI Receive  Priority=2  sciModule=B  dataHead=''  headerCheckMaxCount=16  dataTail=''  dataType=uint8  dataLenOptions=Length via dialog  dataDim=3  maxDataLength=100  initValue=0  errOption=Output custom value  errValue=0  sampleTime=-1  blockingMode=on  timeOut=0.01944  outputStatus=off
      settings: LibrarySourceBlock=c2806xlib/SCI Receive
  Sum2 : Sum  Inputs=|+-
  Sum3 : Sum  Inputs=|+-
  Sum4 : Sum  Inputs=|+-
  Sum5 : Sum  Inputs=|+++  AccumDataTypeStr=double  OutDataTypeStr=double
  y : ArgOut  DisableCoverage=on  ArgumentName=y
  wires:
  Gain2/1 -> Sum5/1
  Demux/2 -> Sum3/1
  Demux/3 -> Sum4/1
  Gain3/1 -> Sum5/2
  Gain4/1 -> Sum5/3
  Demux/1 -> Sum2/1
  Constant3/1 -> Sum3/2
  Sum4/1 -> Gain4/1
  Constant2/1 -> Sum2/2
  Sum2/1 -> Gain2/1
  SCI B Receive/1 -> Demux/1
  Constant4/1 -> Sum4/2
  Sum3/1 -> Gain3/1
  Sum5/1 -> y/1

== system C28069_LLC_ePWM_V8_230307_PhaeShiftWorking/Simulink Function1/Subsystem ==
  In1 : Inport
  Constant : Constant  Value=90E6
  Constant1 : Constant  Value=2
  Divide : Product  Inputs=*/
  Product : Product
  Out1 : Outport
  wires:
  In1/1 -> Product/1
  Constant1/1 -> Product/2
  Constant/1 -> Divide/1
  Product/1 -> Divide/2
  Divide/1 -> Out1/1

== system C28069_LLC_ePWM_V8_230307_PhaeShiftWorking/Softstart @5kHz/GetADC, FaultProtection, SoftStart  @5KHz ==
  note: Old Version Original before/without using case function (Ver. before 19/02/23)
  function : TriggerPort  TriggerType=function-call  VariantControl=(inherit)
  Close Loop Regulation : Subsystem  Commented=on  TreatAsAtomicUnit=on
  Fault Protection @ 5KHz : Subsystem  Commented=on  TreatAsAtomicUnit=on
  Fault Protection @ 5KHz1 : Subsystem  Commented=on  TreatAsAtomicUnit=on
  Frequency Update : Subsystem  Commented=on  TreatAsAtomicUnit=on
  Function-Call Generator : simulink/Ports & Subsystems/Function-Call Generator  Commented=on  sample_time=-1  numberOfIterations=1  DisallowWideOutput=off
  Function-Call Generator1 : simulink/Ports & Subsystems/Function-Call Generator  sample_time=-1  numberOfIterations=1  DisallowWideOutput=off
  Function-Call Split : FunctionCallSplit  Commented=on  IconShape=distinctive  NumOutputPorts=6  OutputPortLayout=default
  Function-Call Split1 : FunctionCallSplit  IconShape=distinctive  NumOutputPorts=6  OutputPortLayout=default
  Get AVG : Subsystem  Commented=on  TreatAsAtomicUnit=on
  SoftStart : Subsystem  Commented=on  TreatAsAtomicUnit=on
  SoftStart1 : Subsystem  TreatAsAtomicUnit=on
  UpdatePWM : Subsystem  Commented=on  TreatAsAtomicUnit=on
  wires:
  Function-Call Generator/1 -> Function-Call Split/1
  Function-Call Split/1 -> Get AVG/Trigger
  Function-Call Split/2 -> Fault Protection @ 5KHz/Trigger
  Function-Call Split/3 -> SoftStart/Trigger
  Function-Call Split/4 -> UpdatePWM/Trigger
  Function-Call Split1/2 -> Fault Protection @ 5KHz1/Trigger
  Function-Call Generator1/1 -> Function-Call Split1/1
  Function-Call Split1/4 -> Close Loop Regulation/Trigger
  Function-Call Split1/5 -> Frequency Update/Trigger
  Function-Call Split1/1 -> SoftStart1/Trigger

== system C28069_LLC_ePWM_V8_230307_PhaeShiftWorking/UART Reporting @ 1Hz/SCI_A_Transmit_function1 ==
  SCI_A_Transmit_VADC_Suffix : TriggerPort  TriggerType=function-call  IsSimulinkFunction=on  FunctionName=SCI_A_Transmit_VADC_Suffix  FunctionVisibility=scoped  VariantControl=(inherit)
  SCI Transmit : c280xlib/SCI Transmit  sciModule=B  dataHead=''  dataTail=10  blockingMode=on  outputStatus=off
  VADC : Constant  Value=[86 65 68 67]  OutDataTypeStr=uint8
  wires:
  VADC/1 -> SCI Transmit/1

== system C28069_LLC_ePWM_V8_230307_PhaeShiftWorking/UART Reporting @ 1Hz/SCI_A_Transmit_function10 ==
  SCI_A_Transmit_VBAT_Suffix : TriggerPort  TriggerType=function-call  IsSimulinkFunction=on  FunctionName=SCI_A_Transmit_VBAT_Suffix  FunctionVisibility=scoped  VariantControl=(inherit)
  SCI Transmit : c280xlib/SCI Transmit  sciModule=A  dataHead=''  dataTail=10  blockingMode=on  outputStatus=off
  VBAT : Constant  Value=[86 66 65 84]  OutDataTypeStr=uint8
  wires:
  VBAT/1 -> SCI Transmit/1

== system C28069_LLC_ePWM_V8_230307_PhaeShiftWorking/UART Reporting @ 1Hz/SCI_A_Transmit_function11 ==
  SCI_A_Transmit_OVPFlag_Suffix : TriggerPort  TriggerType=function-call  IsSimulinkFunction=on  FunctionName=SCI_A_Transmit_OVPFlag_Suffix  FunctionVisibility=scoped  VariantControl=(inherit)
  OVPFlag : Constant  Value=[95 79 86 80 70 108 97 103]  OutDataTypeStr=uint8
  SCI Transmit : c280xlib/SCI Transmit  sciModule=A  dataHead=''  dataTail=10  blockingMode=on  outputStatus=off
  wires:
  OVPFlag/1 -> SCI Transmit/1

== system C28069_LLC_ePWM_V8_230307_PhaeShiftWorking/UART Reporting @ 1Hz/SCI_A_Transmit_function12 ==
  SCI_A_Transmit_Freq_Suffix : TriggerPort  TriggerType=function-call  IsSimulinkFunction=on  FunctionName=SCI_A_Transmit_Freq_Suffix  FunctionVisibility=scoped  VariantControl=(inherit)
  KHz_FreqSend : Constant  Value=[75 72 122 95 70 114 101 113 83 101 110 100]  OutDataTypeStr=uint8
  SCI Transmit : c280xlib/SCI Transmit  sciModule=A  dataHead=''  dataTail=10  blockingMode=on  outputStatus=off
  wires:
  KHz_FreqSend/1 -> SCI Transmit/1

== system C28069_LLC_ePWM_V8_230307_PhaeShiftWorking/UART Reporting @ 1Hz/SCI_A_Transmit_function13 ==
  SCI_A_Transmit_VAvg_Suffix : TriggerPort  TriggerType=function-call  IsSimulinkFunction=on  FunctionName=SCI_A_Transmit_VAvg_Suffix  FunctionVisibility=scoped  VariantControl=(inherit)
  SCI Transmit : c280xlib/SCI Transmit  sciModule=A  dataHead=''  dataTail=10  blockingMode=on  outputStatus=off
  VAvg : Constant  Value=[86 65 118 103]  OutDataTypeStr=uint8
  wires:
  VAvg/1 -> SCI Transmit/1

== system C28069_LLC_ePWM_V8_230307_PhaeShiftWorking/UART Reporting @ 1Hz/SCI_A_Transmit_function14 ==
  SCI_A_Transmit_Vo_Suffix : TriggerPort  TriggerType=function-call  IsSimulinkFunction=on  FunctionName=SCI_A_Transmit_Vo_Suffix  FunctionVisibility=scoped  VariantControl=(inherit)
  SCI Transmit : c280xlib/SCI Transmit  sciModule=A  dataHead=''  dataTail=10  blockingMode=on  outputStatus=off
  Vo : Constant  Value=[86 111]  OutDataTypeStr=uint8
  wires:
  Vo/1 -> SCI Transmit/1

== system C28069_LLC_ePWM_V8_230307_PhaeShiftWorking/UART Reporting @ 1Hz/SCI_A_Transmit_function15 ==
  SCI_A_Transmit_VBAT_Suffix : TriggerPort  TriggerType=function-call  IsSimulinkFunction=on  FunctionName=SCI_A_Transmit_VBAT_Suffix  FunctionVisibility=scoped  VariantControl=(inherit)
  SCI Transmit : c280xlib/SCI Transmit  sciModule=B  dataHead=''  dataTail=10  blockingMode=on  outputStatus=off
  VBAT : Constant  Value=[86 66 65 84]  OutDataTypeStr=uint8
  wires:
  VBAT/1 -> SCI Transmit/1

== system C28069_LLC_ePWM_V8_230307_PhaeShiftWorking/UART Reporting @ 1Hz/SCI_A_Transmit_function16 ==
  SCI_A_Transmit_PFC_Suffix : TriggerPort  TriggerType=function-call  IsSimulinkFunction=on  FunctionName=SCI_A_Transmit_PFC_Suffix  FunctionVisibility=scoped  VariantControl=(inherit)
  PFC : Constant  Value=[80 70 67]  OutDataTypeStr=uint8
  SCI Transmit : c280xlib/SCI Transmit  sciModule=A  dataHead=''  dataTail=10  blockingMode=on  outputStatus=off
  wires:
  PFC/1 -> SCI Transmit/1

== system C28069_LLC_ePWM_V8_230307_PhaeShiftWorking/UART Reporting @ 1Hz/SCI_A_Transmit_function17 ==
  SCI_A_Transmit_Current_Suffix : TriggerPort  TriggerType=function-call  IsSimulinkFunction=on  FunctionName=SCI_A_Transmit_Current_Suffix  FunctionVisibility=scoped  VariantControl=(inherit)
  SCI Transmit : c280xlib/SCI Transmit  sciModule=B  dataHead=''  dataTail=10  blockingMode=on  outputStatus=off
  mA_Iout : Constant  Value=[109 65 95 73 111 117 116]  OutDataTypeStr=uint8
  wires:
  mA_Iout/1 -> SCI Transmit/1

== system C28069_LLC_ePWM_V8_230307_PhaeShiftWorking/UART Reporting @ 1Hz/SCI_A_Transmit_function18 ==
  SCI_A_Transmit_Current_Suffix : TriggerPort  TriggerType=function-call  IsSimulinkFunction=on  FunctionName=SCI_A_Transmit_Current_Suffix  FunctionVisibility=scoped  VariantControl=(inherit)
  SCI Transmit : c280xlib/SCI Transmit  sciModule=A  dataHead=''  dataTail=10  blockingMode=on  outputStatus=off
  mA_Iout : Constant  Value=[109 65 95 73 111 117 116]  OutDataTypeStr=uint8
  wires:
  mA_Iout/1 -> SCI Transmit/1

== system C28069_LLC_ePWM_V8_230307_PhaeShiftWorking/UART Reporting @ 1Hz/SCI_A_Transmit_function19 ==
  SCI_A_Transmit_Duty_Suffix : TriggerPort  TriggerType=function-call  IsSimulinkFunction=on  FunctionName=SCI_A_Transmit_Duty_Suffix  FunctionVisibility=scoped  VariantControl=(inherit)
  Duty : Constant  Value=[68 117 116 121 95 68 66]  OutDataTypeStr=uint8
  SCI Transmit : c280xlib/SCI Transmit  sciModule=B  dataHead=''  dataTail=10  blockingMode=on  outputStatus=off
  wires:
  Duty/1 -> SCI Transmit/1

== system C28069_LLC_ePWM_V8_230307_PhaeShiftWorking/UART Reporting @ 1Hz/SCI_A_Transmit_function2 ==
  SCI_A_Transmit : TriggerPort  TriggerType=function-call  IsSimulinkFunction=on  FunctionName=SCI_A_Transmit  FunctionVisibility=scoped  VariantControl=(inherit)
  Add Constant{,1..4} (5 alike) : Bias  Bias=48  SaturateOnIntegerOverflow=off
  Constant : Constant  Value=10000
  MATLAB Function : MATLAB Function  TreatAsAtomicUnit=on
  Mux : Mux  Inputs=5
  SCI Transmit : c280xlib/SCI Transmit  sciModule=B  dataHead=''  dataTail=''  blockingMode=on  outputStatus=off
  u : ArgIn  DisableCoverage=on  ArgumentName=u
  wires:
  u/1 -> MATLAB Function/1(Main_number)
  Constant/1 -> MATLAB Function/2(Divider)
  MATLAB Function/5(Digit_1) -> Add Constant4/1
  MATLAB Function/4(Digit_2) -> Add Constant3/1
  MATLAB Function/3(Digit_3) -> Add Constant2/1
  MATLAB Function/2(Digit_4) -> Add Constant1/1
  MATLAB Function/1(Digit_5) -> Add Constant/1
  Add Constant/1 -> Mux/1
  Add Constant1/1 -> Mux/2
  Add Constant2/1 -> Mux/3
  Add Constant3/1 -> Mux/4
  Add Constant4/1 -> Mux/5
  Mux/1 -> SCI Transmit/1

== system C28069_LLC_ePWM_V8_230307_PhaeShiftWorking/UART Reporting @ 1Hz/SCI_A_Transmit_function20 ==
  SCI_A_Transmit_Duty_Suffix : TriggerPort  TriggerType=function-call  IsSimulinkFunction=on  FunctionName=SCI_A_Transmit_Duty_Suffix  FunctionVisibility=scoped  VariantControl=(inherit)
  SCI Transmit : c280xlib/SCI Transmit  sciModule=A  dataHead=''  dataTail=10  blockingMode=on  outputStatus=off
  mA_Iout : Constant  Value=[109 65 95 73 111 117 116]  OutDataTypeStr=uint8
  wires:
  mA_Iout/1 -> SCI Transmit/1

== system C28069_LLC_ePWM_V8_230307_PhaeShiftWorking/UART Reporting @ 1Hz/SCI_A_Transmit_function21 ==
  SCI_A_Transmit_VBATRef_Suffix : TriggerPort  TriggerType=function-call  IsSimulinkFunction=on  FunctionName=SCI_A_Transmit_VBATRef_Suffix  FunctionVisibility=scoped  VariantControl=(inherit)
  SCI Transmit : c280xlib/SCI Transmit  sciModule=B  dataHead=''  dataTail=10  blockingMode=on  outputStatus=off
  VBATRef : Constant  Value=[86 66 65 84 82 101 102]  OutDataTypeStr=uint8
  wires:
  VBATRef/1 -> SCI Transmit/1

== system C28069_LLC_ePWM_V8_230307_PhaeShiftWorking/UART Reporting @ 1Hz/SCI_A_Transmit_function22 ==
  SCI_A_Transmit_SS_Suffix : TriggerPort  TriggerType=function-call  IsSimulinkFunction=on  FunctionName=SCI_A_Transmit_SS_Suffix  FunctionVisibility=scoped  VariantControl=(inherit)
  SCI Transmit : c280xlib/SCI Transmit  sciModule=B  dataHead=''  dataTail=10  blockingMode=on  outputStatus=off
  SS : Constant  Value=[83 83]  OutDataTypeStr=uint8
  wires:
  SS/1 -> SCI Transmit/1

== system C28069_LLC_ePWM_V8_230307_PhaeShiftWorking/UART Reporting @ 1Hz/SCI_A_Transmit_function23 ==
  SCI_A_Transmit_TBPHS_Suffix : TriggerPort  TriggerType=function-call  IsSimulinkFunction=on  FunctionName=SCI_A_Transmit_TBPHS_Suffix  FunctionVisibility=scoped  VariantControl=(inherit)
  SCI Transmit : c280xlib/SCI Transmit  sciModule=B  dataHead=''  dataTail=10  blockingMode=on  outputStatus=off
  TBPHS : Constant  Value=[84 66 80 72 83]  OutDataTypeStr=uint8
  wires:
  TBPHS/1 -> SCI Transmit/1

== system C28069_LLC_ePWM_V8_230307_PhaeShiftWorking/UART Reporting @ 1Hz/SCI_A_Transmit_function3 ==
  SCI_A_Transmit_OVPFlag_Suffix : TriggerPort  TriggerType=function-call  IsSimulinkFunction=on  FunctionName=SCI_A_Transmit_OVPFlag_Suffix  FunctionVisibility=scoped  VariantControl=(inherit)
  OVPFlag : Constant  Value=[95 79 86 80 70 108 97 103]  OutDataTypeStr=uint8
  SCI Transmit : c280xlib/SCI Transmit  sciModule=B  dataHead=''  dataTail=10  blockingMode=on  outputStatus=off
  wires:
  OVPFlag/1 -> SCI Transmit/1

== system C28069_LLC_ePWM_V8_230307_PhaeShiftWorking/UART Reporting @ 1Hz/SCI_A_Transmit_function4 ==
  SCI_A_Transmit_VAvg_Suffix : TriggerPort  TriggerType=function-call  IsSimulinkFunction=on  FunctionName=SCI_A_Transmit_VAvg_Suffix  FunctionVisibility=scoped  VariantControl=(inherit)
  SCI Transmit : c280xlib/SCI Transmit  sciModule=B  dataHead=''  dataTail=10  blockingMode=on  outputStatus=off
  VAvg : Constant  Value=[86 65 118 103]  OutDataTypeStr=uint8
  wires:
  VAvg/1 -> SCI Transmit/1

== system C28069_LLC_ePWM_V8_230307_PhaeShiftWorking/UART Reporting @ 1Hz/SCI_A_Transmit_function5 ==
  SCI_A_Transmit_Freq_Suffix : TriggerPort  TriggerType=function-call  IsSimulinkFunction=on  FunctionName=SCI_A_Transmit_Freq_Suffix  FunctionVisibility=scoped  VariantControl=(inherit)
  KHz_FreqSend : Constant  Value=[75 72 122 95 70 114 101 113 83 101 110 100]  OutDataTypeStr=uint8
  SCI Transmit : c280xlib/SCI Transmit  sciModule=B  dataHead=''  dataTail=10  blockingMode=on  outputStatus=off
  wires:
  KHz_FreqSend/1 -> SCI Transmit/1

== system C28069_LLC_ePWM_V8_230307_PhaeShiftWorking/UART Reporting @ 1Hz/SCI_A_Transmit_function6 ==
  SCI_A_Transmit_Vo_Suffix : TriggerPort  TriggerType=function-call  IsSimulinkFunction=on  FunctionName=SCI_A_Transmit_Vo_Suffix  FunctionVisibility=scoped  VariantControl=(inherit)
  SCI Transmit : c280xlib/SCI Transmit  sciModule=B  dataHead=''  dataTail=10  blockingMode=on  outputStatus=off
  Vo : Constant  Value=[86 111]  OutDataTypeStr=uint8
  wires:
  Vo/1 -> SCI Transmit/1

== system C28069_LLC_ePWM_V8_230307_PhaeShiftWorking/UART Reporting @ 1Hz/SCI_A_Transmit_function7 ==
  SCI_A_Transmit_PFC_Suffix : TriggerPort  TriggerType=function-call  IsSimulinkFunction=on  FunctionName=SCI_A_Transmit_PFC_Suffix  FunctionVisibility=scoped  VariantControl=(inherit)
  PFC : Constant  Value=[80 70 67]  OutDataTypeStr=uint8
  SCI Transmit : c280xlib/SCI Transmit  sciModule=B  dataHead=''  dataTail=10  blockingMode=on  outputStatus=off
  wires:
  PFC/1 -> SCI Transmit/1

== system C28069_LLC_ePWM_V8_230307_PhaeShiftWorking/UART Reporting @ 1Hz/SCI_A_Transmit_function8 ==
  SCI_A_Transmit_VADC_Suffix : TriggerPort  TriggerType=function-call  IsSimulinkFunction=on  FunctionName=SCI_A_Transmit_VADC_Suffix  FunctionVisibility=scoped  VariantControl=(inherit)
  SCI Transmit : c280xlib/SCI Transmit  sciModule=A  dataHead=''  dataTail=10  blockingMode=on  outputStatus=off
  VADC : Constant  Value=[86 65 68 67]  OutDataTypeStr=uint8
  wires:
  VADC/1 -> SCI Transmit/1

== system C28069_LLC_ePWM_V8_230307_PhaeShiftWorking/UART Reporting @ 1Hz/SCI_A_Transmit_function9 ==
  SCI_A_Transmit : TriggerPort  TriggerType=function-call  IsSimulinkFunction=on  FunctionName=SCI_A_Transmit  FunctionVisibility=scoped  VariantControl=(inherit)
  Add Constant{,1..4} (5 alike) : Bias  Bias=48  SaturateOnIntegerOverflow=off
  Constant : Constant  Value=10000
  MATLAB Function : MATLAB Function  TreatAsAtomicUnit=on
  Mux : Mux  Inputs=5
  SCI Transmit : c280xlib/SCI Transmit  sciModule=A  dataHead=''  dataTail=''  blockingMode=on  outputStatus=off
  u : ArgIn  DisableCoverage=on  ArgumentName=u
  wires:
  u/1 -> MATLAB Function/1(Main_number)
  Constant/1 -> MATLAB Function/2(Divider)
  MATLAB Function/5(Digit_1) -> Add Constant4/1
  MATLAB Function/4(Digit_2) -> Add Constant3/1
  MATLAB Function/3(Digit_3) -> Add Constant2/1
  MATLAB Function/2(Digit_4) -> Add Constant1/1
  MATLAB Function/1(Digit_5) -> Add Constant/1
  Add Constant/1 -> Mux/1
  Add Constant1/1 -> Mux/2
  Add Constant2/1 -> Mux/3
  Add Constant3/1 -> Mux/4
  Add Constant4/1 -> Mux/5
  Mux/1 -> SCI Transmit/1
